simulink model "BLDC_Demo"  (R2019b)
settings: Solver=FixedStepDiscrete  StartTime=0.0  StopTime=Inf  FixedStep=0.001  RelTol=1e-3  EnableMultiTasking=on
PreLoadFcn:
  | run('BLDC_Demo_ini.m')
PostLoadFcn:
  | , if any(exist('dsrtsu_mdlpostloadfcn', 'file') ~= 0), dsrtsu_mdlpostloadfcn('Execute', bdroot); end,
InitFcn:
  | , if any(exist('rtifpga_mdlclblib', 'file') ~= 0), rtifpga_mdlclblib('Init', bdroot); end,
values from neighbouring files (symbols this model uses):
  BLDC_Ctrl_Ctrl_mode_SW = 3    [BLDC_Demo_ini.m]
  BLDC_Ctrl_iA_Set = 0    [BLDC_Demo_ini.m]
  BLDC_Ctrl_iA_Stroke = 0    [BLDC_Demo_ini.m]
  BLDC_Ctrl_is_dir = is_dir    [BLDC_Demo_ini.m]
  BLDC_Ctrl_is_index = is_index    [BLDC_Demo_ini.m]
  BLDC_Ctrl_Ki_iA = KI_i    (= 7190.04058695)    [BLDC_Demo_ini.m]
  BLDC_Ctrl_Ki_n = KI_n    (= 10.7018628664)    [BLDC_Demo_ini.m]
  BLDC_Ctrl_Kp_iA = KP_i    (= 3.09991410791)    [BLDC_Demo_ini.m]
  BLDC_Ctrl_Kp_n = KP_n    (= 0.0877769226706)    [BLDC_Demo_ini.m]
  BLDC_Ctrl_Limit_iA = IA_MAX    (= 9.5)    [BLDC_Demo_ini.m]
  BLDC_Ctrl_n_Limit = N_MAX    (= 3000)    [BLDC_Demo_ini.m]
  BLDC_Ctrl_n_Set = 0    [BLDC_Demo_ini.m]
  BLDC_Ctrl_n_Stroke = 0    [BLDC_Demo_ini.m]
  BLDC_Ctrl_TF_iA = TF_iA    (= 7.95774715459e-05)    [BLDC_Demo_ini.m]
  BLDC_Ctrl_TF_n = TF_n    (= 0.00159154943092)    [BLDC_Demo_ini.m]
  BLDC_Ctrl_v_Set = 0    [BLDC_Demo_ini.m]
  Modulator_Zi_HSD = Zi_HSD_LSD(:,4:6)    [BLDC_Demo_ini.m]
  Modulator_Zi_LSD = Zi_HSD_LSD(:,7:9)    [BLDC_Demo_ini.m]
  T_PWM = 50e-6    (= 5e-05)    [BLDC_Demo_ini.m]
undefined symbols (not defined in the file or in its folder): clock
libraries: simulink x29, rti1202lib_adc_class1 x8, dsextras x4, rtiemclib x4, rti1202lib_dio_class1 x3, rti1202lib_base x1
(part 3 of 3)

== system BLDC_Demo/Control/Input/min_max_angle ==
  Hall_Signals : Inport
  Bus Selector : BusSelector  OutputSignals=hall_A,hall_B,hall_C
  Math Function : Math  Operator=mod  SaturateOnIntegerOverflow=on
  Math Function1 : Math  Operator=mod  SaturateOnIntegerOverflow=on
  ModValue : Constant  Value=360
  Offset : Constant  Value=-32
  Sum : Sum  Inputs=|++
  Sum1 : Sum  Inputs=|++
  Truth Table : Truth Table  TreatAsAtomicUnit=on
  hall_min : Outport  VectorParamsAs1DForOutWhenUnconnected=off
  hall_max : Outport  Port=2  VectorParamsAs1DForOutWhenUnconnected=off
  wires:
  Hall_Signals/1 -> Bus Selector/1
  Bus Selector/2 -> Truth Table/2(b)  "<hall_B>"
  Bus Selector/3 -> Truth Table/3(c)  "<hall_C>"
  Bus Selector/1 -> Truth Table/1(a)  "<hall_A>"
  Truth Table/1(Min) -> Sum/1
  Truth Table/2(Max) -> Sum1/1
  Offset/1 -> Sum1/2, Sum/2
  Sum/1 -> Math Function/1
  Sum1/1 -> Math Function1/1
  ModValue/1 -> Math Function/2, Math Function1/2
  Math Function/1 -> hall_min/1
  Math Function1/1 -> hall_max/1

== system BLDC_Demo/Control/Output/Calc Phase Duty ==
  Duty : Inport
  Direction : Inport  Port=2
  Position (elec.) : Inport  Port=3
  Calc Sector [1..6] : Subsystem
  Demux : Demux  Outputs=3
  Gain : Gain  Gain=-1
  Mux : Mux  Inputs=3
  Product : Product
  Selector : Selector  InputPortWidth=6  IndexOptions=Starting index (port)  Indices=[1 3]  OutputSizes=1
  Selector1 : Selector  InputPortWidth=6  IndexOptions=Starting index (port)  Indices=[1 3]  OutputSizes=1
  Selector2 : Selector  InputPortWidth=6  IndexOptions=Starting index (port)  Indices=[1 3]  OutputSizes=1
  Switch : Switch  Criteria=u2 > Threshold  Threshold=0.5
  Za : Constant  Value=[1 1 0 -1 -1 0]
  Zb : Constant  Value=[-1 0 1 1 0 -1]
  Zc : Constant  Value=[0 -1 -1 0 1 1]
  Za [-1..1] : Outport  VectorParamsAs1DForOutWhenUnconnected=off
  Zb [-1..1] : Outport  Port=2  VectorParamsAs1DForOutWhenUnconnected=off
  Zc[-1..1] : Outport  Port=3  VectorParamsAs1DForOutWhenUnconnected=off
  wires:
  Position (elec.)/1 -> Calc Sector [1..6]/1(Pos [0..360])
  Calc Sector [1..6]/1(Sector) -> Selector2/2, Selector1/2, Selector/2
  Za/1 -> Selector/1
  Zc/1 -> Selector2/1
  Zb/1 -> Selector1/1
  Selector/1 -> Mux/1
  Selector1/1 -> Mux/2
  Selector2/1 -> Mux/3
  Direction/1 -> Switch/2
  Gain/1 -> Switch/3
  Product/1 -> Switch/1, Gain/1
  Switch/1 -> Demux/1
  Demux/1 -> Za [-1..1]/1
  Demux/2 -> Zb [-1..1]/1
  Demux/3 -> Zc[-1..1]/1
  Mux/1 -> Product/1
  Duty/1 -> Product/2

== system BLDC_Demo/Control/Output/SignalCollector ==
  BusCreator : BusCreator  Inputs=1
  tag scope: BUS_Outputs=global
  wires:
  [PMSM_OUT] -> BusCreator/1
  BusCreator/1 -> [BUS_Outputs]  "Inputs"

== system BLDC_Demo/Control/Output/SignalCollector4 ==
  a : Inport
  b : Inport  Port=2
  c : Inport  Port=3
  Bus Creator : BusCreator  Inputs=3
  SignalBus : Outport  VectorParamsAs1DForOutWhenUnconnected=off
  wires:
  Bus Creator/1 -> SignalBus/1  "Phase_Signals"
  a/1 -> Bus Creator/1  "a"
  b/1 -> Bus Creator/2  "b"
  c/1 -> Bus Creator/3  "c"

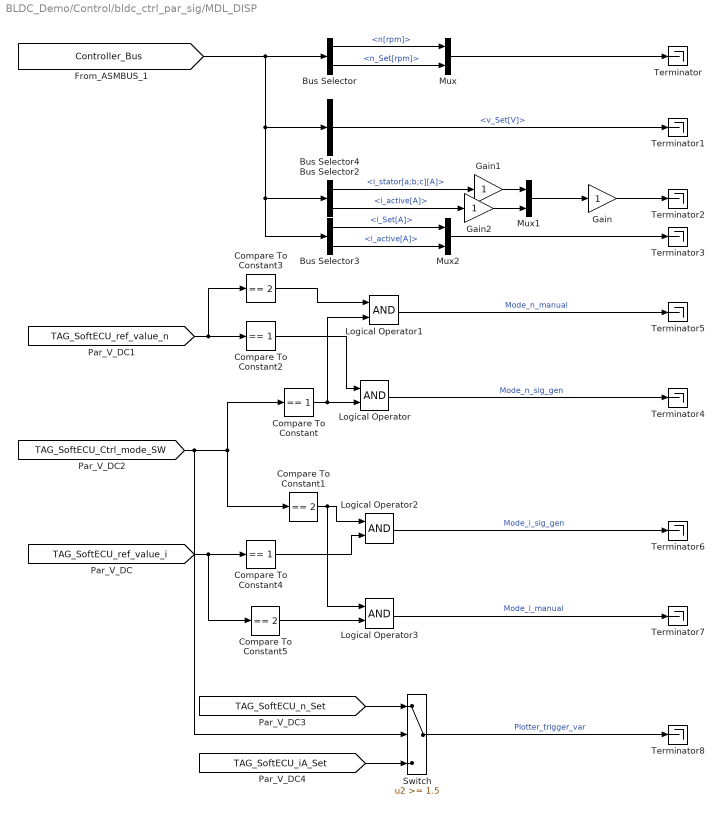
== system BLDC_Demo/Control/bldc_ctrl_par_sig/MDL_DISP ==
  Bus Selector : BusSelector  OutputSignals=BLDC_CONTROLLER.SignalBus_Speed_Controller.n[rpm],BLDC_CONTROLLER.SignalBus_Speed_Controller.n_Set[rpm]
  Bus Selector2 : BusSelector  OutputSignals=BLDC_CONTROLLER.SignalBus_Current_Controller.i_stator[a;b;c][A],BLDC_CONTROLLER.SignalBus_Current_Controller.i_active[A]
  Bus Selector3 : BusSelector  OutputSignals=BLDC_CONTROLLER.SignalBus_Current_Controller.i_Set[A],BLDC_CONTROLLER.SignalBus_Current_Controller.i_active[A]
  Bus Selector4 : BusSelector  OutputSignals=BLDC_CONTROLLER.v_Set[V]
  Compare To Constant : simulink/Logic and Bit Operations/Compare To Constant  relop===  const=1  OutDataTypeStr=uint8  ZeroCross=off
  Compare To Constant1 : simulink/Logic and Bit Operations/Compare To Constant  relop===  const=2  OutDataTypeStr=uint8  ZeroCross=off
  Compare To Constant2 : simulink/Logic and Bit Operations/Compare To Constant  relop===  const=1  OutDataTypeStr=uint8  ZeroCross=off
  Compare To Constant3 : simulink/Logic and Bit Operations/Compare To Constant  relop===  const=2  OutDataTypeStr=uint8  ZeroCross=off
  Compare To Constant4 : simulink/Logic and Bit Operations/Compare To Constant  relop===  const=1  OutDataTypeStr=uint8  ZeroCross=off
  Compare To Constant5 : simulink/Logic and Bit Operations/Compare To Constant  relop===  const=2  OutDataTypeStr=uint8  ZeroCross=off
  Gain : Gain
  Gain1 : Gain
  Gain2 : Gain
  Logical Operator{,1..3} (4 alike) : Logic  AllPortsSameDT=off  OutDataTypeStr=boolean
  Mux : Mux  Inputs=2
  Mux1 : Mux  Inputs=2
  Mux2 : Mux  Inputs=2
  Switch : Switch  Threshold=1.5
  Terminator{,1..8} (9 alike) : Terminator
  wires:
  Mux2/1 -> Terminator3/1
  [Controller_Bus] -> Bus Selector/1, Bus Selector4/1, Bus Selector2/1, Bus Selector3/1
  Bus Selector/1 -> Mux/1  "<n[rpm]>"
  Bus Selector/2 -> Mux/2  "<n_Set[rpm]>"
  Mux/1 -> Terminator/1
  Bus Selector2/1 -> Gain1/1  "<i_stator[a;b;c][A]>"
  Mux1/1 -> Gain/1
  Bus Selector3/1 -> Mux2/1  "<i_Set[A]>"
  Bus Selector3/2 -> Mux2/2  "<i_active[A]>"
  Bus Selector4/1 -> Terminator1/1  "<v_Set[V]>"
  Bus Selector2/2 -> Gain2/1  "<i_active[A]>"
  [TAG_SoftECU_Ctrl_mode_SW] -> Compare To Constant1/1, Compare To Constant/1, Switch/2
  [TAG_SoftECU_ref_value_n] -> Compare To Constant3/1, Compare To Constant2/1
  Compare To Constant/1 -> Logical Operator/2, Logical Operator1/2
  Logical Operator/1 -> Terminator4/1  "Mode_n_sig_gen"
  Compare To Constant2/1 -> Logical Operator/1
  Logical Operator1/1 -> Terminator5/1  "Mode_n_manual"
  Compare To Constant3/1 -> Logical Operator1/1
  Compare To Constant1/1 -> Logical Operator2/1, Logical Operator3/1
  [TAG_SoftECU_ref_value_i] -> Compare To Constant5/1, Compare To Constant4/1
  Compare To Constant4/1 -> Logical Operator2/2
  Logical Operator2/1 -> Terminator6/1  "Mode_i_sig_gen"
  Compare To Constant5/1 -> Logical Operator3/2
  Logical Operator3/1 -> Terminator7/1  "Mode_i_manual"
  [TAG_SoftECU_n_Set] -> Switch/1
  [TAG_SoftECU_iA_Set] -> Switch/3
  Switch/1 -> Terminator8/1  "Plotter_trigger_var"
  Gain/1 -> Terminator2/1
  Gain1/1 -> Mux1/1
  Gain2/1 -> Mux1/2

== system BLDC_Demo/Control/bldc_ctrl_par_sig/MDL_DISP_INPUT ==
  Bus Selector2 : BusSelector  OutputSignals=PMSM_in.Hall_Signals.hall_elec_pos,PMSM_in.Hall_Signals.hall_freqbased_vel,PMSM_in.Hall_Signals.hall_freqbased_vel,PMSM_in.Hall_Signals.hall_signals
  Bus Selector3 : BusSelector  OutputSignals=PMSM_in.ADC_Voltages
  Bus Selector4 : BusSelector  OutputSignals=PMSM_in.Inc_Signals.Inc_mech_pos,PMSM_in.Inc_Signals.Inc_elec_pos,PMSM_in.Inc_Signals.inc_derivative_vel,PMSM_in.Inc_Signals.inc_valid
  Bus to Vector : BusToVector
  Bus to Vector1 : BusToVector
  Mux1 : Mux
  Mux2 : Mux  Inputs=1
  Mux3 : Mux
  Terminator1 : Terminator
  Terminator2 : Terminator
  Terminator3 : Terminator
  wires:
  Mux2/1 -> Terminator3/1
  [BUS_Inputs] -> Bus Selector2/1, Bus Selector3/1, Bus Selector4/1
  Bus Selector2/1 -> Mux1/1  "<hall_elec_pos>"
  Mux1/1 -> Terminator2/1
  Bus Selector3/1 -> Bus to Vector1/1  "<ADC_Voltages>"
  Bus Selector2/2 -> Mux1/2  "<hall_freqbased_vel>"
  Bus Selector4/1 -> Mux3/1  "<Inc_mech_pos>"
  Bus Selector4/2 -> Mux3/2  "<Inc_elec_pos>"
  Mux3/1 -> Terminator1/1
  Bus Selector2/3 -> Mux1/3  "<hall_freqbased_vel>"
  Bus Selector2/4 -> Bus to Vector/1  "<hall_signals>"
  Bus Selector4/4 -> Mux3/4  "<inc_valid>"
  Bus Selector4/3 -> Mux3/3  "<inc_derivative_vel>"
  Bus to Vector/1 -> Mux1/4
  Bus to Vector1/1 -> Mux2/1

== system BLDC_Demo/Control/bldc_ctrl_par_sig/MDL_OUTPUT ==
  Bus Selector : BusSelector  OutputSignals=Phase_Signals.a,Phase_Signals.b,Phase_Signals.c
  Mux : Mux  Inputs=3
  Terminator : Terminator
  wires:
  [BUS_Outputs] -> Bus Selector/1
  Bus Selector/1 -> Mux/1  "<a>"
  Mux/1 -> Terminator/1
  Bus Selector/2 -> Mux/2  "<b>"
  Bus Selector/3 -> Mux/3  "<c>"

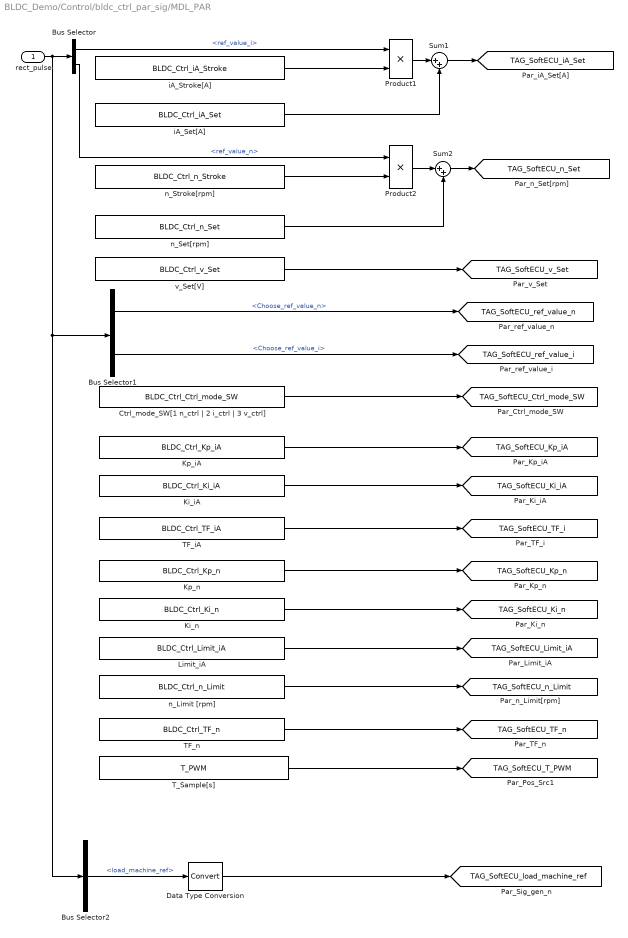
== system BLDC_Demo/Control/bldc_ctrl_par_sig/MDL_PAR ==
  rect_pulse : Inport
  Bus Selector : BusSelector  OutputSignals=ref_value_i,ref_value_n
  Bus Selector1 : BusSelector  OutputSignals=Choose_ref_value_n,Choose_ref_value_i
  Bus Selector2 : BusSelector  OutputSignals=load_machine_ref
  Ctrl_mode_SW[1 n_ctrl | 2 i_ctrl | 3 v_ctrl] : Constant  Value=BLDC_Ctrl_Ctrl_mode_SW
  Data Type Conversion : DataTypeConversion
  Ki_iA : Constant  Value=BLDC_Ctrl_Ki_iA
  Ki_n : Constant  Value=BLDC_Ctrl_Ki_n
  Kp_iA : Constant  Value=BLDC_Ctrl_Kp_iA
  Kp_n : Constant  Value=BLDC_Ctrl_Kp_n
  Limit_iA : Constant  Value=BLDC_Ctrl_Limit_iA
  Product1 : Product  RndMeth=Zero
  Product2 : Product  RndMeth=Zero
  Sum1 : Sum  Inputs=|++
  Sum2 : Sum  Inputs=|++
  TF_iA : Constant  Value=BLDC_Ctrl_TF_iA
  TF_n : Constant  Value=BLDC_Ctrl_TF_n
  T_Sample[s] : Constant  Value=T_PWM
  iA_Set[A] : Constant  Value=BLDC_Ctrl_iA_Set
  iA_Stroke[A] : Constant  Value=BLDC_Ctrl_iA_Stroke
  n_Limit [rpm] : Constant  Value=BLDC_Ctrl_n_Limit
  n_Set[rpm] : Constant  Value=BLDC_Ctrl_n_Set
  n_Stroke[rpm] : Constant  Value=BLDC_Ctrl_n_Stroke
  v_Set[V] : Constant  Value=BLDC_Ctrl_v_Set
  tag scope: TAG_SoftECU_Ctrl_mode_SW=global, TAG_SoftECU_Ki_iA=global, TAG_SoftECU_Ki_n=global, TAG_SoftECU_Kp_iA=global, TAG_SoftECU_Kp_n=global, TAG_SoftECU_Limit_iA=global, TAG_SoftECU_TF_i=global, TAG_SoftECU_TF_n=global, TAG_SoftECU_T_PWM=global, TAG_SoftECU_iA_Set=global, TAG_SoftECU_load_machine_ref=global, TAG_SoftECU_n_Limit=global, TAG_SoftECU_n_Set=global, TAG_SoftECU_ref_value_i=global, TAG_SoftECU_ref_value_n=global, TAG_SoftECU_v_Set=global
  wires:
  Limit_iA/1 -> [TAG_SoftECU_Limit_iA]
  Ki_n/1 -> [TAG_SoftECU_Ki_n]
  Kp_n/1 -> [TAG_SoftECU_Kp_n]
  Ki_iA/1 -> [TAG_SoftECU_Ki_iA]
  Kp_iA/1 -> [TAG_SoftECU_Kp_iA]
  Ctrl_mode_SW[1 n_ctrl | 2 i_ctrl | 3 v_ctrl]/1 -> [TAG_SoftECU_Ctrl_mode_SW]
  v_Set[V]/1 -> [TAG_SoftECU_v_Set]
  n_Limit [rpm]/1 -> [TAG_SoftECU_n_Limit]
  TF_iA/1 -> [TAG_SoftECU_TF_i]
  TF_n/1 -> [TAG_SoftECU_TF_n]
  Product1/1 -> Sum1/1
  Sum1/1 -> [TAG_SoftECU_iA_Set]
  Product2/1 -> Sum2/1
  Sum2/1 -> [TAG_SoftECU_n_Set]
  iA_Set[A]/1 -> Sum1/2
  n_Set[rpm]/1 -> Sum2/2
  iA_Stroke[A]/1 -> Product1/2
  n_Stroke[rpm]/1 -> Product2/2
  rect_pulse/1 -> Bus Selector/1, Bus Selector1/1, Bus Selector2/1
  Bus Selector/1 -> Product1/1  "<ref_value_i>"
  Bus Selector/2 -> Product2/1  "<ref_value_n>"
  T_Sample[s]/1 -> [TAG_SoftECU_T_PWM]
  Bus Selector1/1 -> [TAG_SoftECU_ref_value_n]  "<Choose_ref_value_n>"
  Bus Selector1/2 -> [TAG_SoftECU_ref_value_i]  "<Choose_ref_value_i>"
  Bus Selector2/1 -> Data Type Conversion/1  "<load_machine_ref>"
  Data Type Conversion/1 -> [TAG_SoftECU_load_machine_ref]

== system BLDC_Demo/RTI Data/RTI Data Store/RTI Data Store ==
  RTI Data Store : Subsystem  mask(RTI_DATA_STORE){}
      mask help:
      | RTI Data Store Block. This block is used by RTI to store internal model dependent data. Deleting this block will result in data loss.
      |
      | NEVER DELETE, COPY, OR MODIFY THIS BLOCK!
      mask Help:
      | RTI Data Store Block. This block is used by RTI to store internal model dependent data. Deleting this block will result in data loss.
      | 
      | NEVER DELETE, COPY, OR MODIFY THIS BLOCK!
      mask Display: text(0.5, 0.5, ' ', 'HorizontalAlignment', 'center');

== system BLDC_Demo/Control/Control_load_machine/duty_cycle_2_torque/duty_cycle_2_voltage ==
  In_duty_cycle[0..1] : Inport
  Bus Selector : BusSelector  OutputSignals=ADC_Voltages.Battery_Voltage[V]
  Divide : Product  Inputs=**
  Saturation1 : Saturate  UpperLimit=1  LowerLimit=0
  Out_duty_voltage[V] : Outport  VectorParamsAs1DForOutWhenUnconnected=off
  wires:
  Divide/1 -> Out_duty_voltage[V]/1
  In_duty_cycle[0..1]/1 -> Saturation1/1
  Bus Selector/1 -> Divide/2  "<Battery_Voltage[V]>"
  [BUS_PMSM_IN] -> Bus Selector/1
  Saturation1/1 -> Divide/1

== system BLDC_Demo/Control/Control_load_machine/torque_2_duty_cycle/voltage_2_duty_cycle ==
  In_voltage[V] : Inport
  Bus Selector : BusSelector  OutputSignals=ADC_Voltages.Battery_Voltage[V]
  Divide : Product  Inputs=*/
  Saturation : Saturate  UpperLimit=1  LowerLimit=0
  Out_duty_cycle : Outport  VectorParamsAs1DForOutWhenUnconnected=off
  wires:
  Divide/1 -> Saturation/1
  In_voltage[V]/1 -> Divide/1
  Saturation/1 -> Out_duty_cycle/1
  Bus Selector/1 -> Divide/2  "<Battery_Voltage[V]>"
  [BUS_PMSM_IN] -> Bus Selector/1

== system BLDC_Demo/Control/Control_load_machine/torque_2_duty_cycle1/voltage_2_duty_cycle ==
  In_voltage[V] : Inport
  Bus Selector : BusSelector  OutputSignals=ADC_Voltages.Battery_Voltage[V]
  Divide : Product  Inputs=*/
  Saturation : Saturate  UpperLimit=1  LowerLimit=0
  Out_duty_cycle[0..1] : Outport  VectorParamsAs1DForOutWhenUnconnected=off
  wires:
  [BUS_PMSM_IN] -> Bus Selector/1
  Bus Selector/1 -> Divide/2  "<Battery_Voltage[V]>"
  Saturation/1 -> Out_duty_cycle[0..1]/1
  In_voltage[V]/1 -> Divide/1
  Divide/1 -> Saturation/1

== system BLDC_Demo/Control/Controller/BLDC_CONTROLLER/5x_mean_value ==
  n[rpm] : Inport
  Gain : Gain  Gain=1/5
  Memory{,1..3} (4 alike) : Memory  InheritSampleTime=on
  Sum : Sum  Inputs=+++++
  n_mean[rpm] : Outport  VectorParamsAs1DForOutWhenUnconnected=off
  wires:
  n[rpm]/1 -> Sum/1, Memory/1
  Memory/1 -> Sum/2, Memory1/1
  Memory1/1 -> Sum/3, Memory2/1
  Memory2/1 -> Sum/4, Memory3/1
  Memory3/1 -> Sum/5
  Sum/1 -> Gain/1
  Gain/1 -> n_mean[rpm]/1

== system BLDC_Demo/Control/Controller/BLDC_CONTROLLER/SignalCollector ==
  SignalBus_Speed_Controller : Inport
  V_DCLink[V] : Inport  Port=2
  HallSignal[a;b;c][1|0] : Inport  Port=3
  SignalBus_Current_Controller : Inport  Port=4
  v_Set[V] : Inport  Port=5
  Bus Creator : BusCreator  Inputs=5
  SignalBus : Outport  VectorParamsAs1DForOutWhenUnconnected=off
  wires:
  HallSignal[a;b;c][1|0]/1 -> Bus Creator/5  "HallSignal[a;b;c][0|1]"
  v_Set[V]/1 -> Bus Creator/4  "v_Set[V]"
  V_DCLink[V]/1 -> Bus Creator/3  "V_DCLink[V]"
  Bus Creator/1 -> SignalBus/1  "BLDC_CONTROLLER"
  SignalBus_Speed_Controller/1 -> Bus Creator/1  "SignalBus_Speed_Controller"
  SignalBus_Current_Controller/1 -> Bus Creator/2  "SignalBus_Current_Controller"

== system BLDC_Demo/Control/Controller/BLDC_CONTROLLER/Trigger_250us ==
  Counter Limited : simulink/Sources/Counter Limited  uplimit=4  tsamp=-1
  Lookup Table : Lookup_n-D  NumberOfTableDimensions=1  BreakpointsForDimension1=[0,1,2,3,4]  Table=[1,0,0,0,0]  ExtrapMethod=Clip  InputSameDT=on
  trigger : Outport  VectorParamsAs1DForOutWhenUnconnected=off
  wires:
  Counter Limited/1 -> Lookup Table/1
  Lookup Table/1 -> trigger/1

== system BLDC_Demo/Control/Controller/BLDC_CONTROLLER/current_controller ==
  V_DCLink[V] : Inport
  HallSignal[a;b;c][01] : Inport  Port=2
  i_Set[A] : Inport  Port=3
  Kp_i : Inport  Port=4
  Ki_i : Inport  Port=5
  i_stator[a;b;c][A] : Inport  Port=6
  T_Current_Filter[s] : Inport  Port=7
  T_Sample[s] : Inport  Port=8
  Current_Measurement : Subsystem
  Limit_v_Ctrl : Subsystem
      mask Display: plot([0.15 0.85],[.5 .5],[.5 .5],[0.05 0.95],0.15+0.7*[0 .25 .75 1],0.05+0.9*[.25 .25 .75 .75]);
  PI_CONTROLLER_EXT_SATURATION : Subsystem  mask(PI_CONTROLLER_EXT_SATURATION){ASMProperties=struct('Name','PI_CONTROLLER_EXT_SATURATION','Version','1.0','Library','ASM_ElectricComponents_lib')}
      mask help: (c) Copyright 2007, dSPACE GmbH. All rights reserved.
  SignalCollector : Subsystem
  SignalBus : Outport  VectorParamsAs1DForOutWhenUnconnected=off
  " V_set[V]" : Outport  Port=2  VectorParamsAs1DForOutWhenUnconnected=off
  wires:
  T_Current_Filter[s]/1 -> Current_Measurement/3(T_Current_Filter[s])
  HallSignal[a;b;c][01]/1 -> Current_Measurement/2(HallSignal[a;b;c][0|1])
  i_stator[a;b;c][A]/1 -> SignalCollector/1(i_stator[a;b;c][A]), Current_Measurement/1(i_stator[a;b;c][A])
  T_Sample[s]/1 -> PI_CONTROLLER_EXT_SATURATION/6(T_Sample[s]), Current_Measurement/4(T_Sample[s])
  Current_Measurement/1(i_active[A]) -> PI_CONTROLLER_EXT_SATURATION/1(ActualValue), SignalCollector/2(i_active[A])
  V_DCLink[V]/1 -> Limit_v_Ctrl/2(In2)
  Limit_v_Ctrl/1(Out1) -> PI_CONTROLLER_EXT_SATURATION/5(y_limited), SignalCollector/4(V_Ctrl_lim[V]), " V_set[V]"/1
  Ki_i/1 -> PI_CONTROLLER_EXT_SATURATION/4(Ki)
  Kp_i/1 -> PI_CONTROLLER_EXT_SATURATION/3(Kp)
  PI_CONTROLLER_EXT_SATURATION/1(y) -> Limit_v_Ctrl/1(In1)
  i_Set[A]/1 -> PI_CONTROLLER_EXT_SATURATION/2(RefValue), SignalCollector/3(i_Set[A])
  SignalCollector/1(SignalBus) -> SignalBus/1

== system BLDC_Demo/Control/Controller/BLDC_CONTROLLER/i_set_source_SW ==
  SW : Inport
  i_Set_2 : Inport  Port=2
  i_Set_1 : Inport  Port=3
  i_Limit[A] : Inport  Port=4
  Limit_i_Set : Subsystem
      mask Display: plot([0.15 0.85],[.5 .5],[.5 .5],[0.05 0.95],0.15+0.7*[0 .25 .75 1],0.05+0.9*[.25 .25 .75 .75]);
  Switch : Switch  Threshold=1.5  SaturateOnIntegerOverflow=on
  i_set : Outport  VectorParamsAs1DForOutWhenUnconnected=off
  wires:
  i_Set_1/1 -> Switch/3
  i_Set_2/1 -> Switch/1
  Switch/1 -> Limit_i_Set/1(In1)
  i_Limit[A]/1 -> Limit_i_Set/2(In2)
  Limit_i_Set/1(Out1) -> i_set/1
  SW/1 -> Switch/2

== system BLDC_Demo/Control/Controller/BLDC_CONTROLLER/speed_controller ==
  n[rpm] : Inport
  n_Set[rpm] : Inport  Port=2
  Kp_n : Inport  Port=3
  Ki_n : Inport  Port=4
  i_Limit[A] : Inport  Port=5
  n_Limit[rpm] : Inport  Port=6
  T_Filter[s] : Inport  Port=7
  T_Sample[s] : Inport  Port=8
  Trigger : TriggerPort  VariantControl=Variant
  Constant1 : Constant  Value=0
  Constant2 : Constant
  DISCRETE_PT1 : Subsystem  mask(DISCRETE_PT1){upper_limit_int=struct('v', 1e300), lower_limit_int=struct('v', -1e300), ASMProperties=struct('Name','DISCRETE_PT1','Version','1.0','Library','ASM_ElectricComponents_lib')}
      mask prompts: upper_limit_int "upper limit (Integrator)"; lower_limit_int "lower limit (Integrator)"
      mask help: (c) Copyright 2007, dSPACE GmbH. All rights reserved.
      mask Help: eval(['asm_modelhelp(gcbh)'])
  Gain : Gain  Gain=-1
  Limit_n_Set : Subsystem
      mask Display: plot([0.15 0.85],[.5 .5],[.5 .5],[0.05 0.95],0.15+0.7*[0 .25 .75 1],0.05+0.9*[.25 .25 .75 .75]);
  PI_CONTROLLER : Subsystem  mask(PI_CONTROLLER){ASMProperties=struct('Name','PI_CONTROLLER','Version','1.0','Library','ASM_ElectricComponents_lib')}
      mask help: (c) Copyright 2007, dSPACE GmbH. All rights reserved.
  SignalCollector : Subsystem
  SignalBus : Outport  VectorParamsAs1DForOutWhenUnconnected=off
  I_q_set[A] : Outport  Port=2  VectorParamsAs1DForOutWhenUnconnected=off
  wires:
  SignalCollector/1(SignalBus) -> SignalBus/1
  PI_CONTROLLER/1(y) -> I_q_set[A]/1
  Kp_n/1 -> PI_CONTROLLER/3(Kp)
  Ki_n/1 -> PI_CONTROLLER/4(Ki)
  i_Limit[A]/1 -> PI_CONTROLLER/5(Limit_up), Gain/1
  Gain/1 -> PI_CONTROLLER/6(Limit_lo)
  T_Sample[s]/1 -> PI_CONTROLLER/7(T_Sample[s]), DISCRETE_PT1/5(T_Sample[s])
  Limit_n_Set/1(Out1) -> PI_CONTROLLER/2(RefValue), SignalCollector/2(n_Set[rpm])
  n_Limit[rpm]/1 -> Limit_n_Set/1(In1)
  n_Set[rpm]/1 -> Limit_n_Set/2(In2)
  DISCRETE_PT1/1(Out) -> PI_CONTROLLER/1(ActualValue), SignalCollector/1(n[rpm])
  T_Filter[s]/1 -> DISCRETE_PT1/4(T[s])
  Constant2/1 -> DISCRETE_PT1/3(K)
  Constant1/1 -> DISCRETE_PT1/1(Reset[0|1])
  n[rpm]/1 -> DISCRETE_PT1/2(In)

== system BLDC_Demo/Control/Controller/BLDC_CONTROLLER/v_set_source_SW ==
  SW : Inport
  v_Set_2 : Inport  Port=2
  v_Set_1 : Inport  Port=3
  Switch : Switch  Threshold=2.5  SaturateOnIntegerOverflow=on
  v_Set : Outport  VectorParamsAs1DForOutWhenUnconnected=off
  wires:
  Switch/1 -> v_Set/1
  v_Set_2/1 -> Switch/1
  v_Set_1/1 -> Switch/3
  SW/1 -> Switch/2

== system BLDC_Demo/Control/Controller/BLOCK_MODULATOR/DutyCycle ==
  v_set[V] : Inport
  V_DCLink[V] : Inport  Port=2
  Abs : Abs
  Data Type Conversion : DataTypeConversion
  Product : Product  Inputs=*/  RndMeth=Zero
  Sign : Signum
  d[0_1] : Outport  VectorParamsAs1DForOutWhenUnconnected=off
  DIR : Outport  Port=2  VectorParamsAs1DForOutWhenUnconnected=off
  wires:
  Abs/1 -> d[0_1]/1
  Sign/1 -> DIR/1
  v_set[V]/1 -> Product/1
  V_DCLink[V]/1 -> Product/2
  Product/1 -> Abs/1, Data Type Conversion/1
  Data Type Conversion/1 -> Sign/1

== system BLDC_Demo/Control/Controller/BLOCK_MODULATOR/Label_DutyCycle_HSD[a;b;c][0_1] ==
  In : Inport
  Bus Creator : BusCreator  Inputs=3
  Demux : Demux  Outputs=3
  Out : Outport  VectorParamsAs1DForOutWhenUnconnected=off
  wires:
  In/1 -> Demux/1
  Bus Creator/1 -> Out/1  "DutyCycle_HSD[a;b;c][0_1]"
  Demux/1 -> Bus Creator/1  "DutyCycle_a_HSD[0_1]"
  Demux/2 -> Bus Creator/2  "DutyCycle_b_HSD[0_1]"
  Demux/3 -> Bus Creator/3  "DutyCycle_c_HSD[0_1]"

== system BLDC_Demo/Control/Controller/BLOCK_MODULATOR/Label_DutyCycle_LSD[a;b;c][0_1] ==
  In : Inport
  Bus Creator : BusCreator  Inputs=3
  Demux : Demux  Outputs=3
  Out : Outport  VectorParamsAs1DForOutWhenUnconnected=off
  wires:
  Demux/3 -> Bus Creator/3  "DutyCycle_c_LSD[0_1]"
  Demux/2 -> Bus Creator/2  "DutyCycle_b_LSD[0_1]"
  Demux/1 -> Bus Creator/1  "DutyCycle_a_LSD[0_1]"
  Bus Creator/1 -> Out/1  "DutyCycle_LSD[a;b;c][0_1]"
  In/1 -> Demux/1

== system BLDC_Demo/Control/Controller/BLOCK_MODULATOR/SignalCollector ==
  d[0_1] : Inport
  DIR : Inport  Port=2
  DutyCycle_HSD[a;b;c][0_1] : Inport  Port=3
  DutyCycle_LSD[a;b;c][0_1] : Inport  Port=4
  Bus Creator : BusCreator  Inputs=4
  SignalBus : Outport  VectorParamsAs1DForOutWhenUnconnected=off
  wires:
  DIR/1 -> Bus Creator/4  "DIR"
  d[0_1]/1 -> Bus Creator/3  "d[0_1]"
  DutyCycle_LSD[a;b;c][0_1]/1 -> Bus Creator/2  "DutyCycle_LSD[a;b;c][0_1]"
  DutyCycle_HSD[a;b;c][0_1]/1 -> Bus Creator/1  "DutyCycle_HSD[a;b;c][0_1]"
  Bus Creator/1 -> SignalBus/1  "BLOCK_MODULATOR"

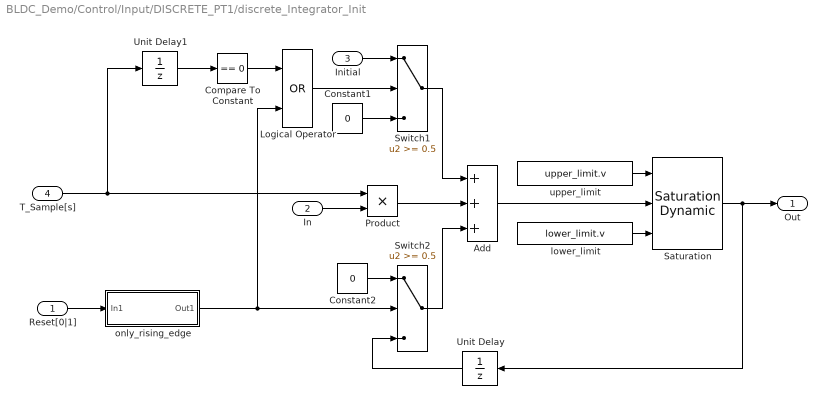
== system BLDC_Demo/Control/Input/DISCRETE_PT1/discrete_Integrator_Init ==
  Reset[0|1] : Inport
  In : Inport  Port=2
  Initial : Inport  Port=3
  T_Sample[s] : Inport  Port=4
  Add : Sum  Inputs=+++
  Compare To Constant : simulink/Logic and Bit Operations/Compare To Constant  relop===  const=0  OutDataTypeStr=uint8  ZeroCross=off
  Constant1 : Constant  Value=0
  Constant2 : Constant  Value=0
  Logical Operator : Logic  Operator=OR  AllPortsSameDT=off  OutDataTypeStr=boolean
  Product : Product  RndMeth=Zero
  Saturation : simulink/Discontinuities/Saturation Dynamic  OutMin=[]  OutMax=[]  OutDataTypeStr=Inherit: Same as second input  OutDataType=sfix(16)  OutScaling=2^-10  DoSatur=off
  Switch1 : Switch  Threshold=0.5
  Switch2 : Switch  Threshold=0.5
  Unit Delay : UnitDelay  SampleTime=-1  HasFrameUpgradeWarning=on
  Unit Delay1 : UnitDelay  SampleTime=-1  HasFrameUpgradeWarning=on
  lower_limit : Constant  Value=lower_limit.v
  "only_rising_edge " : Subsystem
  upper_limit : Constant  Value=upper_limit.v
  Out : Outport  VectorParamsAs1DForOutWhenUnconnected=off
  wires:
  Compare To Constant/1 -> Logical Operator/1
  Logical Operator/1 -> Switch1/2
  Unit Delay1/1 -> Compare To Constant/1
  "only_rising_edge "/1(Out1) -> Switch2/2, Logical Operator/2
  Constant1/1 -> Switch1/3
  Initial/1 -> Switch1/1
  Switch1/1 -> Add/1
  Unit Delay/1 -> Switch2/3
  Switch2/1 -> Add/3
  Constant2/1 -> Switch2/1
  In/1 -> Product/2
  Reset[0|1]/1 -> "only_rising_edge "/1(In1)
  Product/1 -> Add/2
  T_Sample[s]/1 -> Unit Delay1/1, Product/1
  Add/1 -> Saturation/2
  Saturation/1 -> Out/1, Unit Delay/1
  upper_limit/1 -> Saturation/1
  lower_limit/1 -> Saturation/3

== system BLDC_Demo/Control/Output/Calc Phase Duty/Calc Sector [1..6] ==
  Pos [0..360] : Inport
  Math Function : Math  Operator=mod  SaturateOnIntegerOverflow=on
  Sec1 : Constant
  Sec2 : Constant  Value=2
  Sec3 : Constant  Value=3
  Sec4 : Constant  Value=4
  Sec5 : Constant  Value=5
  Sec6 : Constant  Value=6
  Switch : Switch  Criteria=u2 > Threshold  Threshold=300
  Switch1 : Switch  Criteria=u2 > Threshold  Threshold=240
  Switch2 : Switch  Criteria=u2 > Threshold  Threshold=180
  Switch3 : Switch  Criteria=u2 > Threshold  Threshold=120
  Switch4 : Switch  Criteria=u2 > Threshold  Threshold=60
  oneround : Constant  Value=360
  Sector : Outport  VectorParamsAs1DForOutWhenUnconnected=off
  wires:
  Switch2/1 -> Switch1/3
  Switch4/1 -> Switch3/3
  Switch1/1 -> Switch/3
  Switch3/1 -> Switch2/3
  Sec2/1 -> Switch4/1
  Sec1/1 -> Switch4/3
  Sec3/1 -> Switch3/1
  Sec5/1 -> Switch1/1
  Sec4/1 -> Switch2/1
  Sec6/1 -> Switch/1
  Switch/1 -> Sector/1
  Pos [0..360]/1 -> Math Function/1
  Math Function/1 -> Switch4/2, Switch3/2, Switch2/2, Switch/2, Switch1/2
  oneround/1 -> Math Function/2

== system BLDC_Demo/RTI Data/RTI Data Store/RTI Data Store/RTI Data Store ==
  RTI Data Store : Subsystem  mask(RTI_DATA_STORE){}
      mask help:
      | RTI Data Store Block. This block is used by RTI to store internal model dependent data. Deleting this block will result in data loss.
      |
      | NEVER DELETE, COPY, OR MODIFY THIS BLOCK!
      mask Help:
      | RTI Data Store Block. This block is used by RTI to store internal model dependent data. Deleting this block will result in data loss.
      | 
      | NEVER DELETE, COPY, OR MODIFY THIS BLOCK!
      mask Display: text(0.5, 0.5, ' ', 'HorizontalAlignment', 'center');

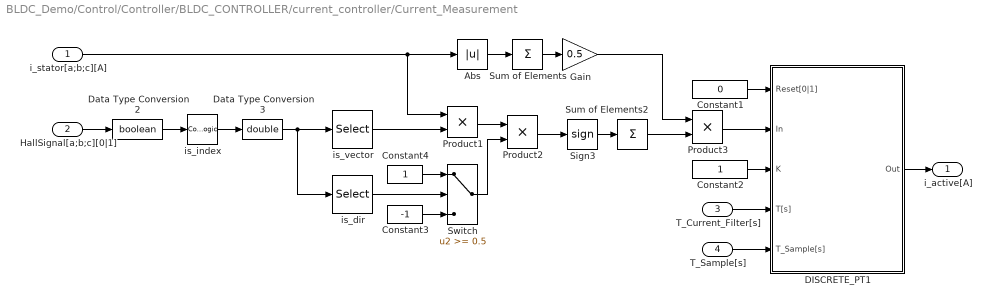
== system BLDC_Demo/Control/Controller/BLDC_CONTROLLER/current_controller/Current_Measurement ==
  i_stator[a;b;c][A] : Inport
  HallSignal[a;b;c][0|1] : Inport  Port=2
  T_Current_Filter[s] : Inport  Port=3
  T_Sample[s] : Inport  Port=4
  Abs : Abs
  Constant1 : Constant  Value=0
  Constant2 : Constant
  Constant3 : Constant  Value=-1
  Constant4 : Constant
  DISCRETE_PT1 : Subsystem  mask(DISCRETE_PT1){upper_limit_int=struct('v', 1e300), lower_limit_int=struct('v', -1e300), ASMProperties=struct('Name','DISCRETE_PT1','Version','1.0','Library','ASM_ElectricComponents_lib')}
      mask prompts: upper_limit_int "upper limit (Integrator)"; lower_limit_int "lower limit (Integrator)"
      mask help: (c) Copyright 2007, dSPACE GmbH. All rights reserved.
      mask Help: eval(['asm_modelhelp(gcbh)'])
  Data Type Conversion2 : DataTypeConversion  OutDataTypeStr=boolean
  Data Type Conversion3 : DataTypeConversion  OutDataTypeStr=double
  Gain : Gain  Gain=0.5
  Product1 : Product  RndMeth=Zero
  Product2 : Product  RndMeth=Zero
  Product3 : Product  RndMeth=Zero
  Sign3 : Signum
  Sum of Elements : Sum  Inputs=+
  Sum of Elements2 : Sum  Inputs=+
  Switch : Switch  Threshold=0.5
  is_dir : Selector  InputPortWidth=4  IndexOptions=Index vector (dialog)  Indices=[4]  OutputSizes=[(-2)]
  is_index : CombinatorialLogic  TruthTable=[is_index, is_dir]
  is_vector : Selector  InputPortWidth=4  IndexOptions=Index vector (dialog)  Indices=[1 2 3]  OutputSizes=[(-2)]
  i_active[A] : Outport  VectorParamsAs1DForOutWhenUnconnected=off
  wires:
  T_Current_Filter[s]/1 -> DISCRETE_PT1/4(T[s])
  Product3/1 -> DISCRETE_PT1/2(In)
  Sum of Elements2/1 -> Product3/2
  Sign3/1 -> Sum of Elements2/1
  Product2/1 -> Sign3/1
  Switch/1 -> Product2/2
  Product1/1 -> Product2/1
  Constant4/1 -> Switch/1
  Constant3/1 -> Switch/3
  is_dir/1 -> Switch/2
  is_vector/1 -> Product1/2
  Data Type Conversion3/1 -> is_dir/1, is_vector/1
  HallSignal[a;b;c][0|1]/1 -> Data Type Conversion2/1
  is_index/1 -> Data Type Conversion3/1
  Data Type Conversion2/1 -> is_index/1
  DISCRETE_PT1/1(Out) -> i_active[A]/1
  Constant2/1 -> DISCRETE_PT1/3(K)
  T_Sample[s]/1 -> DISCRETE_PT1/5(T_Sample[s])
  Constant1/1 -> DISCRETE_PT1/1(Reset[0|1])
  Gain/1 -> Product3/1
  Sum of Elements/1 -> Gain/1
  Abs/1 -> Sum of Elements/1
  i_stator[a;b;c][A]/1 -> Product1/1, Abs/1

== system BLDC_Demo/Control/Controller/BLDC_CONTROLLER/current_controller/Limit_v_Ctrl ==
  In1 : Inport
  In2 : Inport  Port=2
  Saturation Dynamic : simulink/Discontinuities/Saturation Dynamic  OutMin=[]  OutMax=[]  OutDataTypeStr=Inherit: Same as second input  OutDataType=sfix(16)  OutScaling=2^-10  DoSatur=off
  inv : Gain  Gain=-1
  Out1 : Outport  VectorParamsAs1DForOutWhenUnconnected=off
  wires:
  inv/1 -> Saturation Dynamic/3
  In2/1 -> Saturation Dynamic/1, inv/1
  In1/1 -> Saturation Dynamic/2
  Saturation Dynamic/1 -> Out1/1

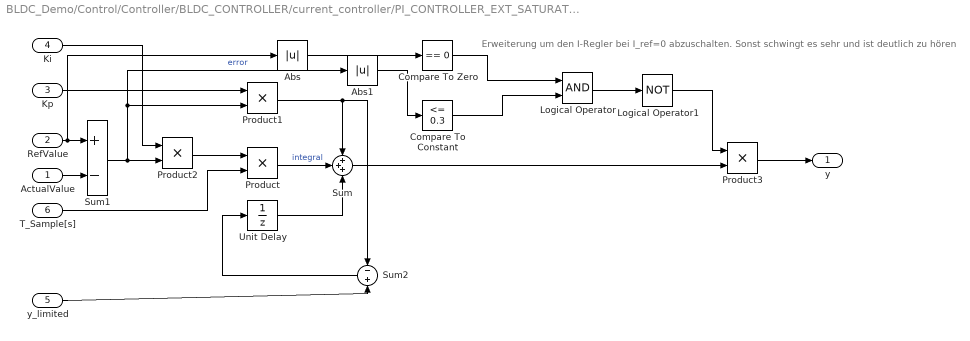
== system BLDC_Demo/Control/Controller/BLDC_CONTROLLER/current_controller/PI_CONTROLLER_EXT_SATURATION ==
  note: Erweiterung um den I-Regler bei I_ref=0 abzuschalten. Sonst schwingt es sehr und ist deutlich zu hören
  ActualValue : Inport
  RefValue : Inport  Port=2
  Kp : Inport  Port=3
  Ki : Inport  Port=4
  y_limited : Inport  Port=5
  T_Sample[s] : Inport  Port=6
  Abs : Abs
  Abs1 : Abs
  Compare To Constant : simulink/Logic and Bit Operations/Compare To Constant  relop=<=  const=0.3  OutDataTypeStr=uint8  ZeroCross=off
  Compare To Zero : simulink/Logic and Bit Operations/Compare To Zero  relop===  OutDataTypeStr=uint8  ZeroCross=off
  Logical Operator : Logic  AllPortsSameDT=off  OutDataTypeStr=boolean
  Logical Operator1 : Logic  Operator=NOT  AllPortsSameDT=off  OutDataTypeStr=boolean
  Product{,1..3} (4 alike) : Product  RndMeth=Zero
  Sum : Sum  Inputs=+++  SaturateOnIntegerOverflow=on
  Sum1 : Sum  Inputs=+-  SaturateOnIntegerOverflow=on
  Sum2 : Sum  Inputs=-|+  SaturateOnIntegerOverflow=on
  Unit Delay : UnitDelay  SampleTime=-1  HasFrameUpgradeWarning=on
  y : Outport  VectorParamsAs1DForOutWhenUnconnected=off
  wires:
  T_Sample[s]/1 -> Product/2
  Sum2/1 -> Unit Delay/1
  Unit Delay/1 -> Sum/3
  Product2/1 -> Product/1
  Sum/1 -> Product3/2
  Product/1 -> Sum/2  "integral"
  Product1/1 -> Sum2/1, Sum/1
  ActualValue/1 -> Sum1/2
  RefValue/1 -> Sum1/1, Abs/1
  Sum1/1 -> Product2/2, Product1/2, Abs1/1  "error"
  y_limited/1 -> Sum2/2
  Kp/1 -> Product1/1
  Ki/1 -> Product2/1
  Compare To Zero/1 -> Logical Operator/1
  Compare To Constant/1 -> Logical Operator/2
  Logical Operator/1 -> Logical Operator1/1
  Product3/1 -> y/1
  Logical Operator1/1 -> Product3/1
  Abs/1 -> Compare To Zero/1
  Abs1/1 -> Compare To Constant/1

== system BLDC_Demo/Control/Controller/BLDC_CONTROLLER/current_controller/SignalCollector ==
  i_stator[a;b;c][A] : Inport
  i_active[A] : Inport  Port=2
  i_Set[A] : Inport  Port=3
  V_Ctrl_lim[V] : Inport  Port=4
  Bus Creator : BusCreator  Inputs=4
  SignalBus : Outport  VectorParamsAs1DForOutWhenUnconnected=off
  wires:
  V_Ctrl_lim[V]/1 -> Bus Creator/4  "V_Ctrl_lim[V]"
  i_active[A]/1 -> Bus Creator/3  "i_active[A]"
  i_Set[A]/1 -> Bus Creator/2  "i_Set[A]"
  i_stator[a;b;c][A]/1 -> Bus Creator/1  "i_stator[a;b;c][A]"
  Bus Creator/1 -> SignalBus/1  "current_controller"

== system BLDC_Demo/Control/Controller/BLDC_CONTROLLER/i_set_source_SW/Limit_i_Set ==
  In1 : Inport
  In2 : Inport  Port=2
  Saturation Dynamic : simulink/Discontinuities/Saturation Dynamic  OutMin=[]  OutMax=[]  OutDataTypeStr=Inherit: Same as second input  OutDataType=sfix(16)  OutScaling=2^-10  DoSatur=off
  inv : Gain  Gain=-1
  Out1 : Outport  VectorParamsAs1DForOutWhenUnconnected=off
  wires:
  Saturation Dynamic/1 -> Out1/1
  In1/1 -> Saturation Dynamic/2
  In2/1 -> inv/1, Saturation Dynamic/1
  inv/1 -> Saturation Dynamic/3

== system BLDC_Demo/Control/Controller/BLDC_CONTROLLER/speed_controller/DISCRETE_PT1 ==
  Reset[0|1] : Inport
  In : Inport  Port=2
  K : Inport  Port=3
  T[s] : Inport  Port=4
  T_Sample[s] : Inport  Port=5
  1|FilterTime : Product  Inputs=*/  SaturateOnIntegerOverflow=on  InputSameDT=on  OutDataTypeStr=Inherit: Same as first input
  Proportional : Product  Inputs=**  SaturateOnIntegerOverflow=on  InputSameDT=on  OutDataTypeStr=Inherit: Same as first input
  Sum : Sum  Inputs=-+|  SaturateOnIntegerOverflow=on  InputSameDT=on  OutDataTypeStr=Inherit: Same as first input
  Unit Delay : UnitDelay  SampleTime=-1  HasFrameUpgradeWarning=on
  discrete_Integrator_Init : Subsystem  mask(DISCRETE_INTEGRATOR){upper_limit=upper_limit_int, lower_limit=lower_limit_int, ASMProperties=struct('Name','discrete_integrator','Version','1.0','Library','ASM_ElectricComponents_lib')}
      mask prompts: upper_limit "upper limit"; lower_limit "lower limit"
      mask help: (c) Copyright 2007, dSPACE GmbH. All rights reserved.
      mask Help: eval(['asm_modelhelp(gcbh)'])
  zero : Constant  Value=0  SampleTime=-1
  Out : Outport  VectorParamsAs1DForOutWhenUnconnected=off
  wires:
  In/1 -> Proportional/1
  Sum/1 -> discrete_Integrator_Init/2(In)
  K/1 -> Proportional/2
  Proportional/1 -> Sum/2
  discrete_Integrator_Init/1(Out) -> 1|FilterTime/1
  1|FilterTime/1 -> Out/1, Unit Delay/1
  Unit Delay/1 -> Sum/1
  T[s]/1 -> 1|FilterTime/2
  Reset[0|1]/1 -> discrete_Integrator_Init/1(Reset[0|1])
  T_Sample[s]/1 -> discrete_Integrator_Init/4(T_Sample[s])
  zero/1 -> discrete_Integrator_Init/3(Initial)

== system BLDC_Demo/Control/Controller/BLDC_CONTROLLER/speed_controller/Limit_n_Set ==
  In1 : Inport
  In2 : Inport  Port=2
  Saturation Dynamic : simulink/Discontinuities/Saturation Dynamic  OutMin=[]  OutMax=[]  OutDataTypeStr=Inherit: Same as second input  OutDataType=sfix(16)  OutScaling=2^-10  DoSatur=off
  inv : Gain  Gain=-1
  Out1 : Outport  VectorParamsAs1DForOutWhenUnconnected=off
  wires:
  inv/1 -> Saturation Dynamic/3
  In2/1 -> Saturation Dynamic/1, inv/1
  In1/1 -> Saturation Dynamic/2
  Saturation Dynamic/1 -> Out1/1

== system BLDC_Demo/Control/Controller/BLDC_CONTROLLER/speed_controller/PI_CONTROLLER ==
  ActualValue : Inport
  RefValue : Inport  Port=2
  Kp : Inport  Port=3
  Ki : Inport  Port=4
  Limit_up : Inport  Port=5
  Limit_lo : Inport  Port=6
  T_Sample[s] : Inport  Port=7
  Product : Product  RndMeth=Zero
  Product1 : Product  RndMeth=Zero
  Product2 : Product  RndMeth=Zero
  Saturation Dynamic : simulink/Discontinuities/Saturation Dynamic  OutMin=[]  OutMax=[]  OutDataTypeStr=Inherit: Same as second input  OutDataType=sfix(16)  OutScaling=2^-10  DoSatur=off
  Sum : Sum  Inputs=+++  SaturateOnIntegerOverflow=on
  Sum1 : Sum  Inputs=+-  SaturateOnIntegerOverflow=on
  Sum2 : Sum  Inputs=-+|  SaturateOnIntegerOverflow=on
  Unit Delay : UnitDelay  SampleTime=-1  HasFrameUpgradeWarning=on
  y : Outport  VectorParamsAs1DForOutWhenUnconnected=off
  wires:
  Limit_lo/1 -> Saturation Dynamic/3
  Limit_up/1 -> Saturation Dynamic/1
  Sum/1 -> Saturation Dynamic/2
  Sum1/1 -> Product1/2, Product2/1  "error"
  RefValue/1 -> Sum1/1
  ActualValue/1 -> Sum1/2
  Product1/1 -> Sum/1, Sum2/1
  Product/1 -> Sum/2  "integral"
  Saturation Dynamic/1 -> Sum2/2, y/1
  Product2/1 -> Product/1
  Unit Delay/1 -> Sum/3
  Sum2/1 -> Unit Delay/1
  T_Sample[s]/1 -> Product/2
  Kp/1 -> Product1/1
  Ki/1 -> Product2/2

== system BLDC_Demo/Control/Controller/BLDC_CONTROLLER/speed_controller/SignalCollector ==
  n[rpm] : Inport
  n_Set[rpm] : Inport  Port=2
  Bus Creator : BusCreator  Inputs=2
  SignalBus : Outport  VectorParamsAs1DForOutWhenUnconnected=off
  wires:
  Bus Creator/1 -> SignalBus/1  "Speed_Controller"
  n_Set[rpm]/1 -> Bus Creator/2  "n_Set[rpm]"
  n[rpm]/1 -> Bus Creator/1  "n[rpm]"

== system BLDC_Demo/Control/Input/DISCRETE_PT1/discrete_Integrator_Init/only_rising_edge  ==
  In1 : Inport
  Compare To Constant1 : simulink/Logic and Bit Operations/Compare To Constant  relop===  const=0  OutDataTypeStr=uint8  ZeroCross=off
  Compare To Constant2 : simulink/Logic and Bit Operations/Compare To Constant  relop===  const=1  OutDataTypeStr=uint8  ZeroCross=off
  Logical Operator1 : Logic  AllPortsSameDT=off  OutDataTypeStr=boolean
  Unit Delay2 : UnitDelay  SampleTime=-1  HasFrameUpgradeWarning=on
  Out1 : Outport  VectorParamsAs1DForOutWhenUnconnected=off
  wires:
  Logical Operator1/1 -> Out1/1
  Compare To Constant2/1 -> Logical Operator1/2
  Compare To Constant1/1 -> Logical Operator1/1
  In1/1 -> Unit Delay2/1, Compare To Constant2/1
  Unit Delay2/1 -> Compare To Constant1/1

== system BLDC_Demo/RTI Data/RTI Data Store/RTI Data Store/RTI Data Store/RTI Data Store ==

== system BLDC_Demo/Control/Controller/BLDC_CONTROLLER/current_controller/Current_Measurement/DISCRETE_PT1 ==
  Reset[0|1] : Inport
  In : Inport  Port=2
  K : Inport  Port=3
  T[s] : Inport  Port=4
  T_Sample[s] : Inport  Port=5
  1|FilterTime : Product  Inputs=*/  SaturateOnIntegerOverflow=on  InputSameDT=on  OutDataTypeStr=Inherit: Same as first input
  Proportional : Product  Inputs=**  SaturateOnIntegerOverflow=on  InputSameDT=on  OutDataTypeStr=Inherit: Same as first input
  Sum : Sum  Inputs=-+|  SaturateOnIntegerOverflow=on  InputSameDT=on  OutDataTypeStr=Inherit: Same as first input
  Unit Delay : UnitDelay  SampleTime=-1  HasFrameUpgradeWarning=on
  discrete_Integrator_Init : Subsystem  mask(DISCRETE_INTEGRATOR){upper_limit=upper_limit_int, lower_limit=lower_limit_int, ASMProperties=struct('Name','discrete_integrator','Version','1.0','Library','ASM_ElectricComponents_lib')}
      mask prompts: upper_limit "upper limit"; lower_limit "lower limit"
      mask help: (c) Copyright 2007, dSPACE GmbH. All rights reserved.
      mask Help: eval(['asm_modelhelp(gcbh)'])
  zero : Constant  Value=0  SampleTime=-1
  Out : Outport  VectorParamsAs1DForOutWhenUnconnected=off
  wires:
  In/1 -> Proportional/1
  Sum/1 -> discrete_Integrator_Init/2(In)
  K/1 -> Proportional/2
  Proportional/1 -> Sum/2
  discrete_Integrator_Init/1(Out) -> 1|FilterTime/1
  1|FilterTime/1 -> Out/1, Unit Delay/1
  Unit Delay/1 -> Sum/1
  T[s]/1 -> 1|FilterTime/2
  Reset[0|1]/1 -> discrete_Integrator_Init/1(Reset[0|1])
  T_Sample[s]/1 -> discrete_Integrator_Init/4(T_Sample[s])
  zero/1 -> discrete_Integrator_Init/3(Initial)

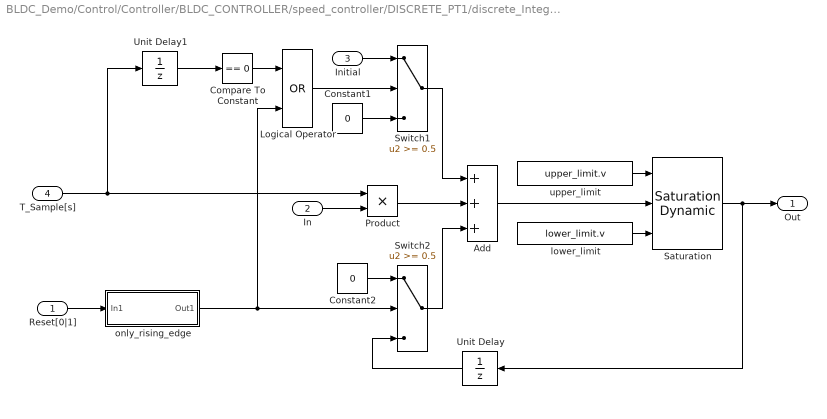
== system BLDC_Demo/Control/Controller/BLDC_CONTROLLER/speed_controller/DISCRETE_PT1/discrete_Integrator_Init ==
  Reset[0|1] : Inport
  In : Inport  Port=2
  Initial : Inport  Port=3
  T_Sample[s] : Inport  Port=4
  Add : Sum  Inputs=+++
  Compare To Constant : simulink/Logic and Bit Operations/Compare To Constant  relop===  const=0  OutDataTypeStr=uint8  ZeroCross=off
  Constant1 : Constant  Value=0
  Constant2 : Constant  Value=0
  Logical Operator : Logic  Operator=OR  AllPortsSameDT=off  OutDataTypeStr=boolean
  Product : Product  RndMeth=Zero
  Saturation : simulink/Discontinuities/Saturation Dynamic  OutMin=[]  OutMax=[]  OutDataTypeStr=Inherit: Same as second input  OutDataType=sfix(16)  OutScaling=2^-10  DoSatur=off
  Switch1 : Switch  Threshold=0.5
  Switch2 : Switch  Threshold=0.5
  Unit Delay : UnitDelay  SampleTime=-1  HasFrameUpgradeWarning=on
  Unit Delay1 : UnitDelay  SampleTime=-1  HasFrameUpgradeWarning=on
  lower_limit : Constant  Value=lower_limit.v
  "only_rising_edge " : Subsystem
  upper_limit : Constant  Value=upper_limit.v
  Out : Outport  VectorParamsAs1DForOutWhenUnconnected=off
  wires:
  Compare To Constant/1 -> Logical Operator/1
  Logical Operator/1 -> Switch1/2
  Unit Delay1/1 -> Compare To Constant/1
  "only_rising_edge "/1(Out1) -> Switch2/2, Logical Operator/2
  Constant1/1 -> Switch1/3
  Initial/1 -> Switch1/1
  Switch1/1 -> Add/1
  Unit Delay/1 -> Switch2/3
  Switch2/1 -> Add/3
  Constant2/1 -> Switch2/1
  In/1 -> Product/2
  Reset[0|1]/1 -> "only_rising_edge "/1(In1)
  Product/1 -> Add/2
  T_Sample[s]/1 -> Unit Delay1/1, Product/1
  Add/1 -> Saturation/2
  Saturation/1 -> Out/1, Unit Delay/1
  upper_limit/1 -> Saturation/1
  lower_limit/1 -> Saturation/3

== system BLDC_Demo/Control/Controller/BLDC_CONTROLLER/current_controller/Current_Measurement/DISCRETE_PT1/discrete_Integrator_Init ==
  Reset[0|1] : Inport
  In : Inport  Port=2
  Initial : Inport  Port=3
  T_Sample[s] : Inport  Port=4
  Add : Sum  Inputs=+++
  Compare To Constant : simulink/Logic and Bit Operations/Compare To Constant  relop===  const=0  OutDataTypeStr=uint8  ZeroCross=off
  Constant1 : Constant  Value=0
  Constant2 : Constant  Value=0
  Logical Operator : Logic  Operator=OR  AllPortsSameDT=off  OutDataTypeStr=boolean
  Product : Product  RndMeth=Zero
  Saturation : simulink/Discontinuities/Saturation Dynamic  OutMin=[]  OutMax=[]  OutDataTypeStr=Inherit: Same as second input  OutDataType=sfix(16)  OutScaling=2^-10  DoSatur=off
  Switch1 : Switch  Threshold=0.5
  Switch2 : Switch  Threshold=0.5
  Unit Delay : UnitDelay  SampleTime=-1  HasFrameUpgradeWarning=on
  Unit Delay1 : UnitDelay  SampleTime=-1  HasFrameUpgradeWarning=on
  lower_limit : Constant  Value=lower_limit.v
  "only_rising_edge " : Subsystem
  upper_limit : Constant  Value=upper_limit.v
  Out : Outport  VectorParamsAs1DForOutWhenUnconnected=off
  wires:
  Compare To Constant/1 -> Logical Operator/1
  Logical Operator/1 -> Switch1/2
  Unit Delay1/1 -> Compare To Constant/1
  "only_rising_edge "/1(Out1) -> Switch2/2, Logical Operator/2
  Constant1/1 -> Switch1/3
  Initial/1 -> Switch1/1
  Switch1/1 -> Add/1
  Unit Delay/1 -> Switch2/3
  Switch2/1 -> Add/3
  Constant2/1 -> Switch2/1
  In/1 -> Product/2
  Reset[0|1]/1 -> "only_rising_edge "/1(In1)
  Product/1 -> Add/2
  T_Sample[s]/1 -> Unit Delay1/1, Product/1
  Add/1 -> Saturation/2
  Saturation/1 -> Out/1, Unit Delay/1
  upper_limit/1 -> Saturation/1
  lower_limit/1 -> Saturation/3

== system BLDC_Demo/Control/Controller/BLDC_CONTROLLER/speed_controller/DISCRETE_PT1/discrete_Integrator_Init/only_rising_edge  ==
  In1 : Inport
  Compare To Constant1 : simulink/Logic and Bit Operations/Compare To Constant  relop===  const=0  OutDataTypeStr=uint8  ZeroCross=off
  Compare To Constant2 : simulink/Logic and Bit Operations/Compare To Constant  relop===  const=1  OutDataTypeStr=uint8  ZeroCross=off
  Logical Operator1 : Logic  AllPortsSameDT=off  OutDataTypeStr=boolean
  Unit Delay2 : UnitDelay  SampleTime=-1  HasFrameUpgradeWarning=on
  Out1 : Outport  VectorParamsAs1DForOutWhenUnconnected=off
  wires:
  Logical Operator1/1 -> Out1/1
  Compare To Constant2/1 -> Logical Operator1/2
  Compare To Constant1/1 -> Logical Operator1/1
  In1/1 -> Unit Delay2/1, Compare To Constant2/1
  Unit Delay2/1 -> Compare To Constant1/1

== system BLDC_Demo/Control/Controller/BLDC_CONTROLLER/current_controller/Current_Measurement/DISCRETE_PT1/discrete_Integrator_Init/only_rising_edge  ==
  In1 : Inport
  Compare To Constant1 : simulink/Logic and Bit Operations/Compare To Constant  relop===  const=0  OutDataTypeStr=uint8  ZeroCross=off
  Compare To Constant2 : simulink/Logic and Bit Operations/Compare To Constant  relop===  const=1  OutDataTypeStr=uint8  ZeroCross=off
  Logical Operator1 : Logic  AllPortsSameDT=off  OutDataTypeStr=boolean
  Unit Delay2 : UnitDelay  SampleTime=-1  HasFrameUpgradeWarning=on
  Out1 : Outport  VectorParamsAs1DForOutWhenUnconnected=off
  wires:
  Logical Operator1/1 -> Out1/1
  Compare To Constant2/1 -> Logical Operator1/2
  Compare To Constant1/1 -> Logical Operator1/1
  In1/1 -> Unit Delay2/1, Compare To Constant2/1
  Unit Delay2/1 -> Compare To Constant1/1

== matlab function BLDC_Demo/Control/Input/min_max_angle/Truth Table ==
  data: a input; Min output; b input; c input; Max output double
function [Min, Max] = fcn(a, b, c)

aVarTruthTableCondition_1 = false;
aVarTruthTableCondition_2 = false;
aVarTruthTableCondition_3 = false;
aVarTruthTableCondition_4 = false;
aVarTruthTableCondition_5 = false;
aVarTruthTableCondition_6 = false;


% Sector 1

aVarTruthTableCondition_1 = logical(a == 1 && b == 0 && c == 1);

% Sector 2

aVarTruthTableCondition_2 = logical(a == 1 && b == 0 && c == 0);

% Sector 3

aVarTruthTableCondition_3 = logical(a == 1 && b == 1 && c == 0);

% Sector 4

aVarTruthTableCondition_4 = logical(a == 0 && b == 1 && c == 0);

% Sector 5

aVarTruthTableCondition_5 = logical(a == 0 && b == 1 && c == 1);

% Sector 6

aVarTruthTableCondition_6 = logical(a == 0 && b == 0 && c == 1);

if (aVarTruthTableCondition_1 && ~aVarTruthTableCondition_2 && ~aVarTruthTableCondition_3 && ~aVarTruthTableCondition_4 && ~aVarTruthTableCondition_5 && ~aVarTruthTableCondition_6)
    aFcnTruthTableAction_1();
elseif (~aVarTruthTableCondition_1 && aVarTruthTableCondition_2 && ~aVarTruthTableCondition_3 && ~aVarTruthTableCondition_4 && ~aVarTruthTableCondition_5 && ~aVarTruthTableCondition_6)
    aFcnTruthTableAction_2();
elseif (~aVarTruthTableCondition_1 && ~aVarTruthTableCondition_2 && aVarTruthTableCondition_3 && ~aVarTruthTableCondition_4 && ~aVarTruthTableCondition_5 && ~aVarTruthTableCondition_6)
    aFcnTruthTableAction_3();
elseif (~aVarTruthTableCondition_1 && ~aVarTruthTableCondition_2 && ~aVarTruthTableCondition_3 && aVarTruthTableCondition_4 && ~aVarTruthTableCondition_5 && ~aVarTruthTableCondition_6)
    aFcnTruthTableAction_4();
elseif (~aVarTruthTableCondition_1 && ~aVarTruthTableCondition_2 && ~aVarTruthTableCondition_3 && ~aVarTruthTableCondition_4 && aVarTruthTableCondition_5 && ~aVarTruthTableCondition_6)
    aFcnTruthTableAction_5();
elseif (~aVarTruthTableCondition_1 && ~aVarTruthTableCondition_2 && ~aVarTruthTableCondition_3 && ~aVarTruthTableCondition_4 && ~aVarTruthTableCondition_5 && aVarTruthTableCondition_6)
    aFcnTruthTableAction_6();
else % Default
    aFcnTruthTableAction_7();
end

function aFcnTruthTableAction_1()

% Sector 1

Min = 0;
Max = 60;

function aFcnTruthTableAction_2()

% Sector 2

Min = 60;
Max = 120;

function aFcnTruthTableAction_3()

% Sector 3

Min = 120;
Max = 180;

function aFcnTruthTableAction_4()

% Sector 4

Min = 180;
Max = 240;

function aFcnTruthTableAction_5()

% Sector 5

Min = 240;
Max = 300;

function aFcnTruthTableAction_6()

% Sector 6

Min = 300;
Max = 360;

function aFcnTruthTableAction_7()

% Invalid

Min = -1;
Max = -1;
